simulink model "two_states_with_two_substates_variant_13"  (R2017b)
settings: Solver=FixedStepDiscrete  StartTime=0.0  StopTime=10.0  RelTol=1e-3
libraries: simulink x1
settings Model: Creator=flosch  LastModifiedBy=flosch
settings OptimizationCC: DefaultParameterBehavior=Inlined  UseDivisionForNetSlopeComputation=on  UseFloatMulNetSlope=on  InlineInvariantSignals=on  PassReuseOutputArgsAs=Individual arguments  ZeroExternalMemoryAtStartup=off  ZeroInternalMemoryAtStartup=off  NoFixptDivByZeroProtection=on  EfficientFloat2IntCast=on  LifeSpan=1
settings DebuggingCC: ParameterTunabilityLossMsg=error
settings HardwareCC: ProdBitPerLong=64  ProdLongLongMode=on  ProdHWDeviceType=Intel->x86-64 (Linux 64)
settings SFSimCC: MATLABDynamicMemAlloc=off
settings RTWCC: SystemTargetFile=ert.tlc  TemplateMakefile=ert_default_tmf  GenerateReport=on  IncludeHyperlinkInReport=on  LaunchReport=on  GenerateTraceInfo=on  GenerateTraceReport=on  GenerateTraceReportSl=on  GenerateTraceReportSf=on  GenerateTraceReportEml=on  GenerateCodeMetricsReport=on
settings CodeAppCC: ForceParamTrailComments=on  IgnoreCustomStorageClasses=off  OperatorAnnotations=on  SimulinkDataObjDesc=on  SFDataObjDesc=on  CustomSymbolStrGlobalVar=rt$N$M  CustomSymbolStrType=$N$M  CustomSymbolStrFcn=$N$M$F  CustomSymbolStrMacro=$N$M  InsertBlockDesc=on
settings ERTTargetCC: TargetLangStandard=C99 (ISO)  GenerateSampleERTMain=on  IncludeMdlTerminateFcn=off  CombineSignalStateStructs=on  SupportAbsoluteTime=off  SupportComplex=off  SupportNonInlinedSFcns=on  InlinedParameterPlacement=NonHierarchical  ERTCustomFileTemplate=example_file_process.tlc  ERTFilePackagingFormat=CompactWithDataFile
settings ConfigComp: CovScope=ReferencedModels  CovIncludeTopModel=off

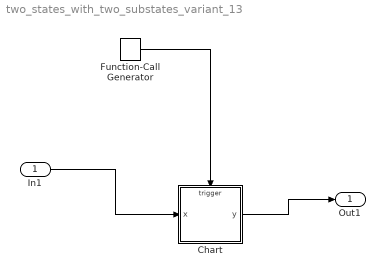
== system two_states_with_two_substates_variant_13 ==
  In1 : Inport
  Chart : Stateflow chart  TreatAsAtomicUnit=on
  Function-Call Generator : simulink/Ports & Subsystems/Function-Call Generator  sample_time=1  numberOfIterations=1
  Out1 : Outport
  wires:
  Function-Call Generator/1 -> Chart/Trigger
  In1/1 -> Chart/1(x)
  Chart/1(y) -> Out1/1

== stateflow chart two_states_with_two_substates_variant_13/Chart ==
  settings: executeAtInitialization=1
  state Big_Kitten
    state Spork
      entry: y = 4;
    state Kitten
      entry: y = 0;
    state Spud
      entry: y = 5;
    state Potato
      entry: y = 1;
    (default) -> Kitten
    Spud -> Spork : Event_B
    Kitten -> Potato : Event_B
    Potato -> Spud : Event_B
  state Big_Potato
    state Tango
      entry: y = x - 1;
    state Fish
      entry: y = 2;
    state Mango
      entry: y = x + 1;
    state Horse
      entry: y = x;
    state Lemon
      entry: y = -x;
    (default) -> Fish
    Fish -> Tango [order 1] : Event_B [x == 1]
    Fish -> Mango [order 2] : Event_B [x == 0]
    Fish -> Lemon [order 4] : Event_B [x < 0]
    Fish -> Horse [order 3] : Event_B [x > 0]
    Mango -> Lemon : Event_B
  note: cyc = 32
      | obj = 26
      | lines = 25
  state Wibble
    entry: y = 3;
  (default) -> Big_Kitten
  Big_Potato -> Big_Kitten : Event_A
  Big_Kitten -> Wibble : Event_A
  Wibble -> Big_Potato : Event_A
  data: x input; y output
  events: Event_A input FUNCTION_CALL_EVENT; Event_B input FUNCTION_CALL_EVENT
